simulink model "V_REP_SIMULINK"  (R2014a)
settings: Solver=FixedStepDiscrete  StartTime=0.0  StopTime=100.0  FixedStep=0.01  RelTol=1e-3
undefined symbols (not defined in the file or in its folder): DiscIntNeverNeededParam, gray
libraries: visionsinks x1
settings Model: Creator=Iseberg  LastModifiedBy=Iseberg

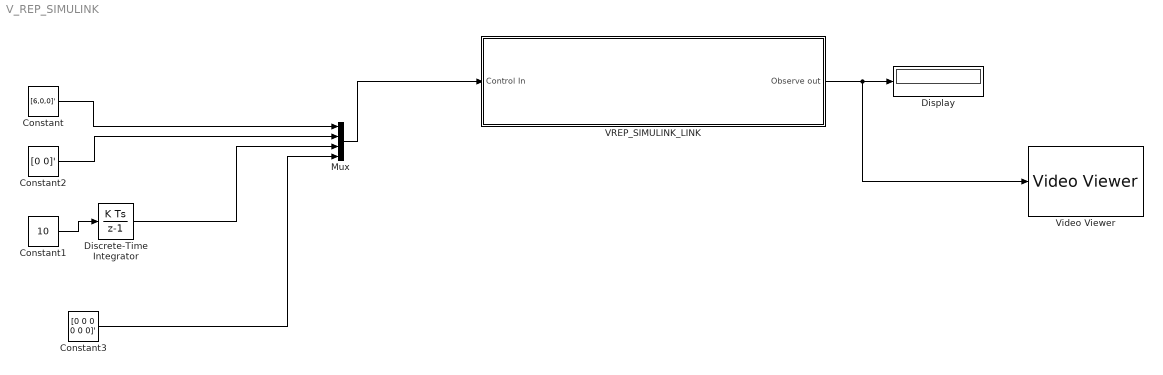
== system V_REP_SIMULINK ==
  Constant : Constant  Value=[6,0,0]'  SampleTime=0.01
  Constant1 : Constant  Value=10
  Constant2 : Constant  Value=[0 0]'  SampleTime=0.01
  Constant3 : Constant  Value=[0 0 0 0 0 0]'  SampleTime=0.01
  Discrete-Time Integrator : DiscreteIntegrator  SampleTime=0.01  ICPrevOutput=DiscIntNeverNeededParam  ICPrevScaledInput=DiscIntNeverNeededParam
  Display : Display
  Mux : Mux
  VREP_SIMULINK_LINK : Subsystem  mask{ObjectsInScene=DefaultCamera, m_ControlObjects={ 'Satellite_Model','Parent';'Satellite_Model_Est','Parent'}, m_InitialControllablePose={zeros(1,6);zeros(1,6)}, m_ObserveObjects={ 'Vision_sensor','Image' }, sceneFileName=C:\Program Files (x86)\V-REP3\V-REP_PRO_EDU\scenes\Scene_MotionEstimation.ttt, OutPortSampleTime=0.05}
      mask prompts: ObjectsInScene "Objects present in scene:"; m_ControlObjects "Control Objects:"; m_InitialControllablePose "Initial Pose:"; m_ObserveObjects "Observing Objects:"; sceneFileName "Scene filename:"; OutPortSampleTime "VREP Sample time [s]"
      mask TypeOptions ObjectsInScene: DefaultCamera | DefaultXViewCamera | DefaultYViewCamera | DefaultZViewCamera | XYZCameraProxy | DefaultNXViewCamera | DefaultNYViewCamera | DefaultNZViewCamera | DefaultLightA | DefaultLightB | DefaultLightC | DefaultLightD | ResizableFloor_5_25 | ResizableFloor_5_25_element | ResizableFloor_5_25_visibleElement | Satellite_Model | redundantRobot | redundantRob_manipSphere | redundantRob_target | redundantRob_link0 | redundantRob_joint1 | Rectangle | redundantRob_joint2 | Cylinder1 | redundantRob_joint3 | Rectangle2 | redundantRob_joint4 | Cylinder2 | redundantRob_joint5 | Rectangle3 | redundantRob_joint6 | Cylinder3 | redundantRob_joint7 | Rectangle4 | redundantRob_link7 | redundantRob_tip | redundantRob_link6 | redundantRob_link5 | redundantRob_link4 | redundantRob_link3 | redundantRob_link2 | redundantRob_link1 | Vision_sensor | Satellite_Model_Est
      mask TypeOptions m_ControlObjects: VREP_SIMULINK_SYS_OBJ/m_ControlObjects
      mask TypeOptions m_InitialControllablePose: VREP_SIMULINK_SYS_OBJ/m_InitialControllablePose
      mask TypeOptions m_ObserveObjects: VREP_SIMULINK_SYS_OBJ/m_ObserveObjects
      mask TypeOptions sceneFileName: VREP_SIMULINK_SYS_OBJ/sceneFileName
      mask TypeOptions OutPortSampleTime: Rate Transition/OutPortSampleTime | Rate Transition1/OutPortSampleTime
      mask DialogControl Control1 Prompt: V-REP Simulink LINK block settings
      mask DialogControl Container8 Prompt: V-REP settings
      mask Display:
      | image('C:\Users\Iseberg\Pictures\Vrep_image.png')
      | port_label('input',1,'Control in');
      | port_label('output',1,'Observe out');
  Video Viewer : visionsinks/Video Viewer  inputType=Obsolete7b  imagePorts=One multidimensional signal  useColorMap=off  colormapValue=gray(256)  specRange=off  minInputVal=0  maxInputVal=255  FigPos=[1 726 1366 627]  AxisZoom=on  trueSizedOnce=off  OpenAtMdlStart=on  DefaultConfigurationName=vipscopes.VideoViewerScopeCfg
  wires:
  VREP_SIMULINK_LINK/1(Observe out) -> Video Viewer/1, Display/1
  Constant1/1 -> Discrete-Time Integrator/1
  Constant/1 -> Mux/1
  Constant2/1 -> Mux/2
  Discrete-Time Integrator/1 -> Mux/3
  Mux/1 -> VREP_SIMULINK_LINK/1(Control In)
  Constant3/1 -> Mux/4

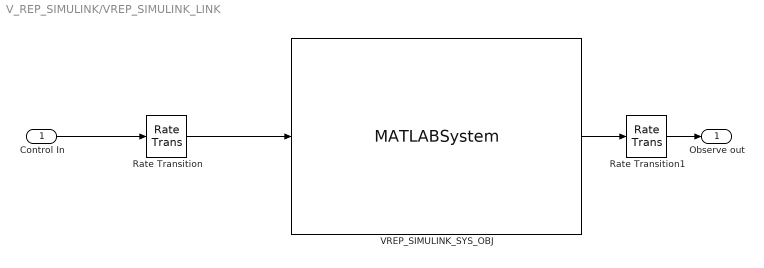
== system V_REP_SIMULINK/VREP_SIMULINK_LINK ==
  Control In : Inport
  Rate Transition : RateTransition  OutPortSampleTime=OutPortSampleTime
  Rate Transition1 : RateTransition  OutPortSampleTime=OutPortSampleTime
  VREP_SIMULINK_SYS_OBJ : MATLABSystem  System=SysObjVREP_1  SimulateUsing=Interpreted execution  ObjectsInScene=''  sceneFileName=C:\Program Files (x86)\V-REP3\V-REP_PRO_EDU\scenes\Scene_MotionEstimation.ttt  m_ControlObjects=m_ControlObjects  m_ObserveObjects=m_ObserveObjects  m_InitialControllablePose=m_InitialControllablePose
      mask Type: SysObjVREP_1
      mask Display:
      | disp('V-REP');
      | port_label('input',1,'ControlPose(2)');
      | port_label('output',1,'ObservePose(1)');
  Observe out : Outport
  wires:
  Control In/1 -> Rate Transition/1
  VREP_SIMULINK_SYS_OBJ/1 -> Rate Transition1/1
  Rate Transition/1 -> VREP_SIMULINK_SYS_OBJ/1
  Rate Transition1/1 -> Observe out/1
